simulink model "HapticPaddle2015b"  (Simulink 8.6)
settings: Solver=ode4  StartTime=0.0  StopTime=10.0  FixedStep=0.01  RelTol=1e-3
values from neighbouring files (symbols this model uses):
  B_eq = B_p + B_m * R^2    (= 0.00017775)    [main.m]
  g = 9.81    [main.m]
  J_eq = J_p + (J_rotor+J_m) * R^2    (= 0.0005755)    [main.m]
  l = 0.0199    [main.m]
  m_p = 0.075    [main.m]
  R = r_p1 / r_m    (= 15)    [main.m]
  r_p2 = 0.065    [main.m]
libraries: simulink_extras x3
settings Model: Creator=jemetzge  LastModifiedBy=Romain
settings DebuggingCC: FcnCallInpInsideContextMsg=EnableAllAsWarning  AllowSymbolicDim=on
settings ConfigComp: CovSFcnEnable=off

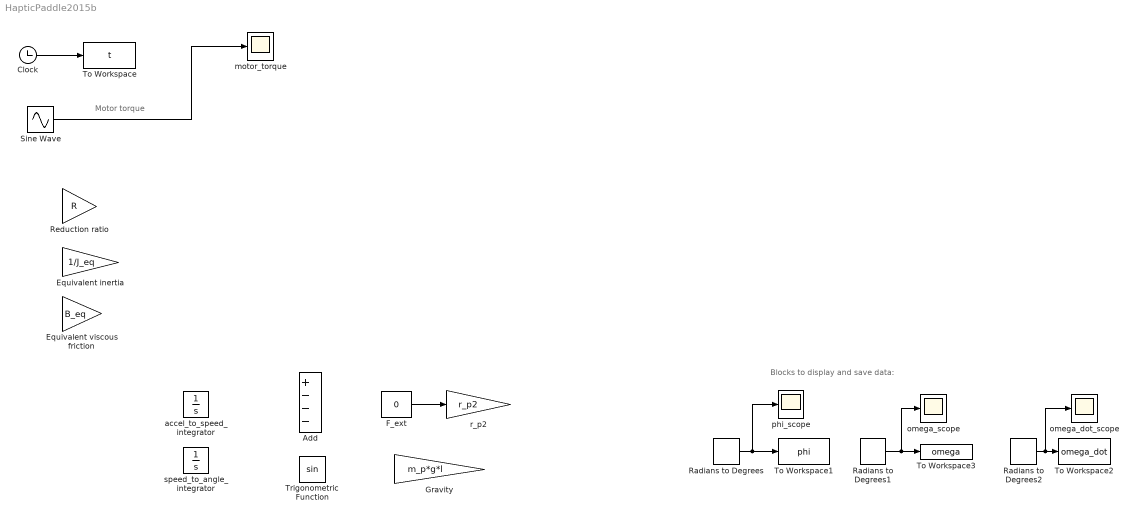
== system HapticPaddle2015b ==
  note: Motor torque
  note: Blocks to display and save data:
  Add : Sum  Inputs=+---
  Clock : Clock
  Equivalent inertia : Gain  Gain=1/J_eq
  Equivalent viscous friction : Gain  Gain=B_eq
  F_ext : Constant  Value=0
  Gravity : Gain  Gain=m_p*g*l
  Radians to Degrees : simulink_extras/Transformations/Radians to Degrees
  Radians to Degrees1 : simulink_extras/Transformations/Radians to Degrees
  Radians to Degrees2 : simulink_extras/Transformations/Radians to Degrees
  Reduction ratio : Gain  Gain=R
  Sine Wave : Sin  Amplitude=0.001  Frequency=2*pi*0.5  SampleTime=0
  To Workspace : ToWorkspace  VariableName=t  SampleTime=-1
  To Workspace1 : ToWorkspace  VariableName=phi  SampleTime=-1
  To Workspace2 : ToWorkspace  VariableName=omega_dot  SampleTime=-1
  To Workspace3 : ToWorkspace  VariableName=omega  SampleTime=-1
  Trigonometric Function : Trigonometry
  accel_to_speed_integrator : Integrator
  motor_torque : Scope
  omega_dot_scope : Scope
  omega_scope : Scope
  phi_scope : Scope
  r_p2 : Gain  Gain=r_p2
  speed_to_angle_integrator : Integrator
  wires:
  F_ext/1 -> r_p2/1
  Radians to Degrees/1 -> phi_scope/1, To Workspace1/1
  Clock/1 -> To Workspace/1
  Radians to Degrees1/1 -> omega_scope/1, To Workspace3/1
  Sine Wave/1 -> motor_torque/1
  Radians to Degrees2/1 -> omega_dot_scope/1, To Workspace2/1
